simulink model "Runge_Kutta_Localization"  (R2024b)
settings: Solver=VariableStepAuto  StartTime=0.0  StopTime=10.0  RelTol=1e-3
values from neighbouring files (symbols this model uses):
  x0 = zeros(10, 1)    [Planning_Adaptive_LTV.m]
undefined symbols (not defined in the file or in its folder): p, Ts
settings Model: Creator=chiar_zjcy1by  LastModifiedBy=chiar_zjcy1by

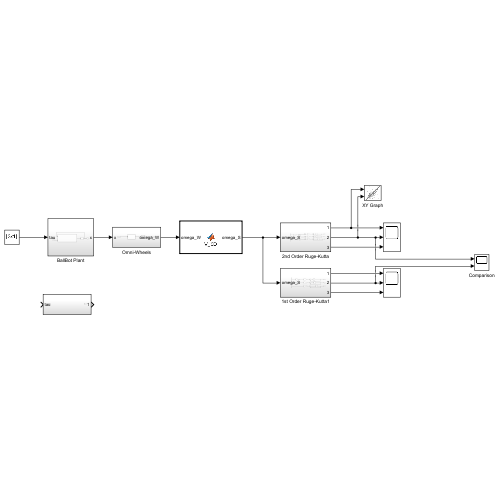
[thumbnail: Simulink's stored preview of the top-level diagram]
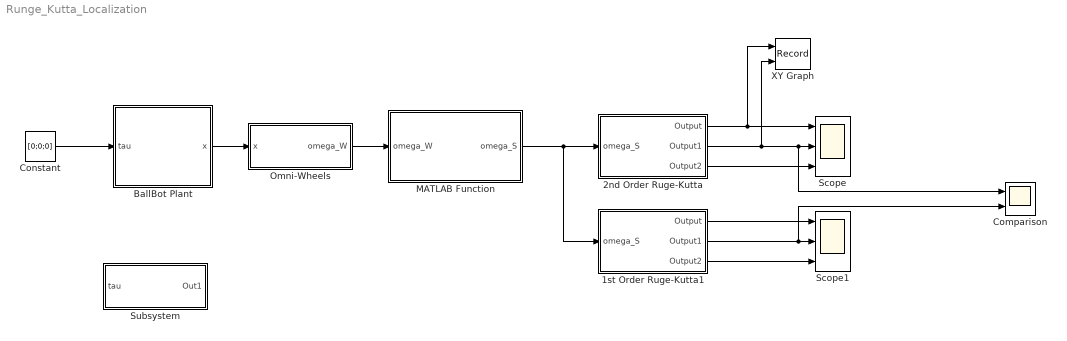
== system Runge_Kutta_Localization ==
  1st Order Ruge-Kutta1 : Subsystem
  2nd Order Ruge-Kutta : Subsystem
  BallBot Plant : Subsystem
  Comparison : Scope  NumInputPorts=2
  Constant : Constant  Value=[0;0;0]
  MATLAB Function : MATLAB Function  TreatAsAtomicUnit=on
  Omni-Wheels : Subsystem
  Scope : Scope  NumInputPorts=3
  Scope1 : Scope  NumInputPorts=3
  Subsystem : Subsystem
  XY Graph : Record  FileSettingsInternal="{\"entries\":[{\"content\":{\"excelSettings\":{\"content\":{},\"type\":\"Streamout.ExcelSettings\"}},\"type\":\"Streamout.FileSettingStorage\",\"uuid\":\"\"}],\"packageUris\":[\"http:\\/\\/schema.mathworks.com\\/mf0\\/streamout_blocks\\/R2020a\"],\"version\":\"1.0\"}"  Layout=[1 1]  SignalsInternal="{\"entries\":[{\"content\":{\"signals\":[{\"content\":{\"blockPath\":[],\"dimensions\":[1],\"domain\":\"\",\"lineColor\":\"#a2142f\",\"plots\":[ 1 ],\"port\":1,\"signalID\":1,\"signalName\":\"2nd Order Ruge-Kutta:1\"},\"type\":\"RecordBlkView.Signal\",\"uuid\":\"\"},{\"content\":{\"blockPath\":[],\"dimensions\":[1],\"domain\":\"\",\"lineColor\":\"#139fff\",\"plots\":[ 1 ],\"port\":2,\"signalID\":2,\"signalName\":\"2nd Order Ruge-Kutta:2\"},\"type\":\"RecordBlkView.Signal\",\"uuid\":\"\"}]},\"type\":\"RecordBlkView.InputSignals\",\"uuid\":\"\"}],\"packageUris\":[\"http:\\/\\/schema.mathworks.com\\/mf0\\/streamout_blocks\\/R2020a\"],\"version\":\"1.0\"}"  VisualizationBindings="{\"xyplotplugin\":{\"info\":[{\"series\":[{\"bindingParametersList\":[{\"parameter\":\"X-Axis\",\"signalID\":1,\"signalName\":\"2nd Order Ruge-Kutta:1\"},{\"parameter\":\"Y-Axis\",\"signalID\":2,\"signalName\":\"2nd Order Ruge-Kutta:2\"}],\"seriesID\":0}],\"subplotID\":1}]}}"  CompatibilityTag=XY
  wires:
  BallBot Plant/1(x) -> Omni-Wheels/1(x)
  Omni-Wheels/1(omega_W) -> MATLAB Function/1(omega_W)
  Constant/1 -> BallBot Plant/1(tau)
  MATLAB Function/1(omega_S) -> 1st Order Ruge-Kutta1/1(omega_S), 2nd Order Ruge-Kutta/1(omega_S)
  2nd Order Ruge-Kutta/1(Output) -> XY Graph/1, Scope/1
  2nd Order Ruge-Kutta/2(Output1) -> XY Graph/2, Comparison/1, Scope/2
  2nd Order Ruge-Kutta/3(Output2) -> Scope/3
  1st Order Ruge-Kutta1/1(Output) -> Scope1/1
  1st Order Ruge-Kutta1/2(Output1) -> Comparison/2, Scope1/2
  1st Order Ruge-Kutta1/3(Output2) -> Scope1/3

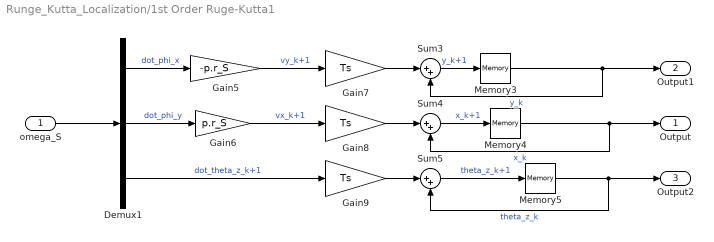
== system Runge_Kutta_Localization/1st Order Ruge-Kutta1 ==
  omega_S : Inport
  Demux1 : Demux  Outputs=3
  Gain5 : Gain  Gain=-p.r_S
  Gain6 : Gain  Gain=p.r_S
  Gain7 : Gain  Gain=Ts
  Gain8 : Gain  Gain=Ts
  Gain9 : Gain  Gain=Ts
  Memory3 : Memory
  Memory4 : Memory
  Memory5 : Memory
  Sum3 : Sum  Inputs=|++
  Sum4 : Sum  Inputs=|++
  Sum5 : Sum  Inputs=|++
  Output : Outport
  Output1 : Outport  Port=2
  Output2 : Outport  Port=3
  wires:
  Gain7/1 -> Sum3/1
  Memory3/1 -> Sum3/2, Output1/1  "y_k"
  Gain8/1 -> Sum4/1
  omega_S/1 -> Demux1/1
  Demux1/1 -> Gain5/1  "dot_phi_x"
  Memory4/1 -> Sum4/2, Output/1  "x_k"
  Sum4/1 -> Memory4/1  "x_k+1"
  Sum3/1 -> Memory3/1  "y_k+1"
  Gain6/1 -> Gain8/1  "vx_k+1"
  Gain9/1 -> Sum5/1
  Memory5/1 -> Output2/1, Sum5/2  "theta_z_k"
  Sum5/1 -> Memory5/1  "theta_z_k+1"
  Gain5/1 -> Gain7/1  "vy_k+1"
  Demux1/2 -> Gain6/1  "dot_phi_y"
  Demux1/3 -> Gain9/1  "dot_theta_z_k+1"

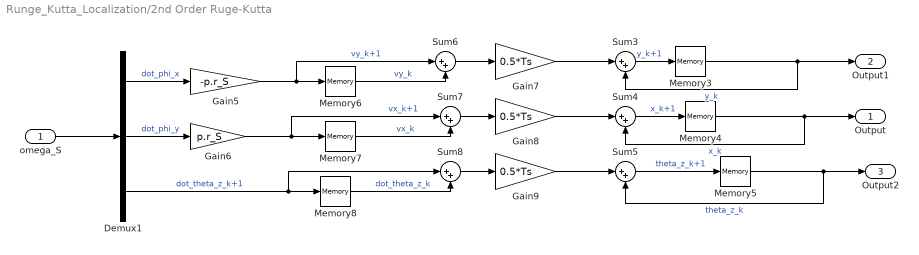
== system Runge_Kutta_Localization/2nd Order Ruge-Kutta ==
  omega_S : Inport
  Demux1 : Demux  Outputs=3
  Gain5 : Gain  Gain=-p.r_S
  Gain6 : Gain  Gain=p.r_S
  Gain7 : Gain  Gain=0.5*Ts
  Gain8 : Gain  Gain=0.5*Ts
  Gain9 : Gain  Gain=0.5*Ts
  Memory{3..8} (6 alike) : Memory
  Sum{3..8} (6 alike) : Sum  Inputs=|++
  Output : Outport
  Output1 : Outport  Port=2
  Output2 : Outport  Port=3
  wires:
  Demux1/3 -> Sum8/1, Memory8/1  "dot_theta_z_k+1"
  Demux1/2 -> Gain6/1  "dot_phi_y"
  Gain5/1 -> Sum6/1, Memory6/1  "vy_k+1"
  Sum6/1 -> Gain7/1
  Memory7/1 -> Sum7/2  "vx_k"
  Sum5/1 -> Memory5/1  "theta_z_k+1"
  Memory8/1 -> Sum8/2  "dot_theta_z_k"
  Memory5/1 -> Output2/1, Sum5/2  "theta_z_k"
  Gain9/1 -> Sum5/1
  Gain6/1 -> Sum7/1, Memory7/1  "vx_k+1"
  Sum3/1 -> Memory3/1  "y_k+1"
  Sum4/1 -> Memory4/1  "x_k+1"
  Memory4/1 -> Output/1, Sum4/2  "x_k"
  Memory6/1 -> Sum6/2  "vy_k"
  Demux1/1 -> Gain5/1  "dot_phi_x"
  Sum7/1 -> Gain8/1
  omega_S/1 -> Demux1/1
  Gain8/1 -> Sum4/1
  Sum8/1 -> Gain9/1
  Memory3/1 -> Output1/1, Sum3/2  "y_k"
  Gain7/1 -> Sum3/1

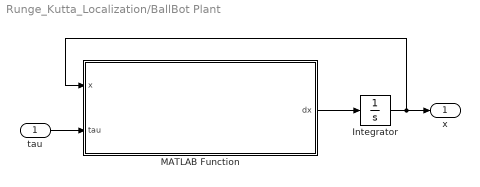
== system Runge_Kutta_Localization/BallBot Plant ==
  tau : Inport
  Integrator : Integrator  InitialCondition=x0(1:10)
  MATLAB Function : MATLAB Function  TreatAsAtomicUnit=on
  x : Outport
  wires:
  MATLAB Function/1(dx) -> Integrator/1
  Integrator/1 -> MATLAB Function/1(x), x/1
  tau/1 -> MATLAB Function/2(tau)

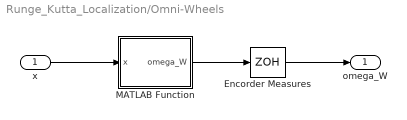
== system Runge_Kutta_Localization/Omni-Wheels ==
  x : Inport
  Encorder Measures : ZeroOrderHold  SampleTime=Ts
  MATLAB Function : MATLAB Function  TreatAsAtomicUnit=on
  omega_W : Outport
  wires:
  x/1 -> MATLAB Function/1(x)
  Encorder Measures/1 -> omega_W/1
  MATLAB Function/1(omega_W) -> Encorder Measures/1

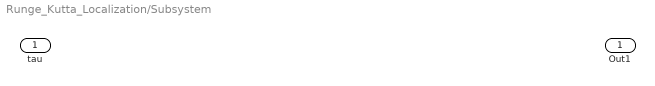
== system Runge_Kutta_Localization/Subsystem ==
  tau : Inport
  Out1 : Outport

== matlab function Runge_Kutta_Localization/MATLAB Function ==
  data: omega_S output; omega_W input; p parameter
function omega_S = V_3D (omega_W, p)
%alpha is the angular displacement of the contact point with the vertical axis of the sphere wheel. 
%beta is the vector of the angual displacements of each omni-wheel qith
%respect to the x axis of the sphere wheel and those are [0, 2*pi/3,4*pi/3]

alpha = pi/4; % alpha = p.alpha;
beta = [0; 2*pi/2; 4*pi/3];% beta = p.beta;
r_S = p.r_S;
r_W = p.r_ow;

    M = zeros(3,3);
    for i=1:length(beta)
        Rot_mat = Rot_z(beta(i))*Rot_y(alpha);
        
        e_Wz = Rot_mat(:,3);
        e_Wy = Rot_mat(:,2);
        e_Wx = Rot_mat(:,1);
        
        M(i,:) = cross(e_Wz,e_Wy)';       
    end
    omega_S = r_W/r_S *(inv(M)*omega_W);
end

function Rz = Rot_z(ang)
    Rz = [cos(ang) -sin(ang) 0;
          sin(ang)  cos(ang) 0;
          0 0 1];
end

function Rx = Rot_x(ang)
    Rx = [1 0 0;
          0 cos(ang) -sin(ang);
          0 sin(ang)  cos(ang);];
end

function Ry = Rot_y(ang)
    Ry = [cos(ang),  0, sin(ang);
          0,         1, 0;
         -sin(ang), 0, cos(ang)];
end

== matlab function Runge_Kutta_Localization/Omni-Wheels/MATLAB Function ==
  data: omega_W output; x input; p parameter

function omega_W = V_3D_inv (x, p)
% alpha is the angular displacement of the contact point with the vertical axis of the sphere wheel.
alpha = pi/4; % alpha = p.alpha;
beta = [0; 2*pi/2; 4*pi/3];% beta = p.beta;
r_S = p.r_S;
r_W = p.r_ow;
% beta is the vector of the angual displacements of each omni-wheel qith
%respect to the x axis of the sphere wheel and those are [0, 2*pi/3,4*pi/3]
    phi_x = x(9);
    phi_y = x(10);
    
    omega_S = [phi_x phi_y  0]';
    M = zeros(3,3);
    
        for i=1:length(beta)
        Rot_mat = Rot_z(beta(i))*Rot_y(alpha);
        
        e_Wz = Rot_mat(:,3);
        e_Wy = Rot_mat(:,2);
        e_Wx = Rot_mat(:,1);
        
        M(i,:) = cross(e_Wz,e_Wy)';    
           
        end
    omega_W = r_S/r_W * M * omega_S;
end

function Rz = Rot_z(ang)
 Rz = [cos(ang) -sin(ang) 0;
      sin(ang)  cos(ang) 0;
      0 0 1];
end

function Rx = Rot_x(ang)
 Rx = [1 0 0;
      0 cos(ang) -sin(ang);
      0 sin(ang)  cos(ang)];
end

function Ry = Rot_y(ang)
    Ry = [cos(ang),  0, sin(ang);
          0,         1, 0;
         -sin(ang), 0, cos(ang)];
end

== matlab function Runge_Kutta_Localization/BallBot Plant/MATLAB Function ==
  data: dx output; x input; p parameter; tau input
function dx = stateDerivative3D_generated(x, p, tau)
    % SW was assumed to not spin relative to the ground
    
    % Unpack state vector (10 elements)
    theta_x = x(1); dot_theta_x = x(6);
    theta_y = x(2); dot_theta_y = x(7);
    theta_z = x(3); dot_theta_z = x(8);
    % phi_x   = x(4); % Not needed for dynamics
    % phi_y   = x(5); % Not needed for dynamics
    dot_phi_x   = x(9);
    dot_phi_y   = x(10);
    
    % Unpack input torques
    tau_x = tau(1);
    tau_y = tau(2);
    tau_z = tau(3);

    % --- Prepare arguments for auto-generated functions ---
    % Argument list for parameters (order MUST match the generator script)
    params_arg = [p.m_U, p.I_Uy, p.I_Ux, p.l_U, p.m_S, p.I_S, p.r_S, p.g, p.b_theta, p.b_phi];

    % --- X-Z Plane (Roll) Dynamics ---
    states_arg_x = [theta_x, dot_theta_x, dot_phi_x];
    inputs_arg_x = [tau_x];
    ddot_theta_x = autogen_ddot_theta_x(states_arg_x, inputs_arg_x, params_arg);
    ddot_phi_x   = autogen_ddot_phi_x(states_arg_x, inputs_arg_x, params_arg);

    % --- Y-Z Plane (Pitch) Dynamics ---
    states_arg_y = [theta_y, dot_theta_y, dot_phi_y];
    inputs_arg_y = [tau_y];
    ddot_theta_y = autogen_ddot_theta_y(states_arg_y, inputs_arg_y, params_arg);
    ddot_phi_y   = autogen_ddot_phi_y(states_arg_y, inputs_arg_y, params_arg);
    
    % --- Transversal Plane Dynamics (Yaw) ---
    % Using the simple decoupled model from your original script
    ddot_theta_z = (tau_z - p.fz * dot_theta_z) / p.Iz;
    
    % --- Assemble the state derivative vector dx ---
    dx = [
        dot_theta_x;    % dx(1) = d(theta_x)/dt
        dot_theta_y;    % dx(2) = d(theta_y)/dt
        dot_theta_z;    % dx(3) = d(theta_z)/dt
        dot_phi_x;      % dx(4) = d(phi_x)/dt
        dot_phi_y;      % dx(5) = d(phi_y)/dt
        ddot_theta_x;   % dx(6) = d(dot_theta_x)/dt
        ddot_theta_y;   % dx(7) = d(dot_theta_y)/dt
        ddot_theta_z;   % dx(8) = d(dot_theta_z)/dt
        ddot_phi_x;     % dx(9) = d(dot_phi_x)/dt
        ddot_phi_y;     % dx(10)= d(dot_phi_y)/dt
    ];
end
